simulink model "Base"  (R2023b)
settings: Solver=ode3  StartTime=0.0  StopTime=inf  RelTol=1e-3  EnableMultiTasking=on
PreLoadFcn:
  | addpath(genpath('AS5600_Driver'))
  | addpath(genpath('Servo_Driver'))
  | addpath(genpath('Wattmeter_INA219_Driver'))
libraries: arduinolib x6, arduinosensorlib x2
settings Model: FPTRunName=Active  SimulationMode=external  ExtModeTrigDuration=2  Creator=Rafael  LastModifiedBy=Rafael
settings SolverCC: AlgebraicLoopSolver=TrustRegion  AutoInsertRateTranBlk=on
settings DataIOCC: LimitDataPoints=on  SaveFormat=Array
settings OptimizationCC: ReuseModelBlockBuffer=off  ExpressionDepthLimit=2147483647  LifeSpan=Inf  MaxStackSize=64
settings DebuggingCC: UnderspecifiedInitializationDetection=Classic  MergeDetectMultiDrivingBlocksExec=none  FcnCallInpInsideContextMsg=warning  UnconnectedInputMsg=warning  UnconnectedOutputMsg=warning  UnconnectedLineMsg=warning  AllowSymbolicDim=off  StateNameClashWarn=warning  SFUnexpectedBacktrackingDiag=warning  SFNoUnconditionalDefaultTransitionDiag=warning  SFExecutionAtInitializationDiag=none  ArithmeticOperatorsInVariantConditions=warning
settings HardwareCC: ProdBitPerPointer=32  ProdBitPerSizeT=32  ProdBitPerPtrDiffT=32  ProdLargestAtomicInteger=Long  ProdLargestAtomicFloat=Double  ProdWordSize=32  ProdHWDeviceType=ARM Compatible->ARM Cortex
settings ModelReferenceCC: EnableRefExpFcnMdlSchedulingChecks=on  PropagateSignalLabelsOutOfModel=off
settings SFSimCC: SimUseLocalCustomCode=off  CustomCodeUndefinedFunction=UseInterfaceOnly
settings RTWCC: Description=Embedded Coder  SystemTargetFile=ert.tlc  HardwareBoard=Arduino Due  TemplateMakefile=ert_default_tmf  GenerateReport=on  RTWVerbose=off  RTWUseLocalCustomCode=off  Toolchain=Arduino ARM  BuildConfiguration=Faster Runs  LaunchReport=on
settings CodeAppCC: ForceParamTrailComments=on  OperatorAnnotations=on  StateflowObjectComments=on  MATLABSourceComments=on
settings ERTTargetCC: MultiwordLength=2048  ERTCustomFileBanners=off  SupportContinuousTime=on  SupportNonInlinedSFcns=on  RemoveResetFunc=off  SupportVariableSizeSignals=on  ModelStepFunctionPrototypeControlCompliant=off  ExtMode=on  ExtModeTransport=3  ExtModeStaticAlloc=on  ExtModeAutomaticAllocSize=off  ExtModeStaticAllocSize=24576  ExtModeMexFile=ext_xcp  ExtModeMexArgs=0 4 115200  ExtModeIntrfLevel=Level2 - Open
settings ConfigComp: CovMetricSettings=dw  CovSaveCumulativeToWorkspaceVar=on  CovSaveSingleToWorkspaceVar=on  CovExternalEMLEnable=off  CovSFcnEnable=off

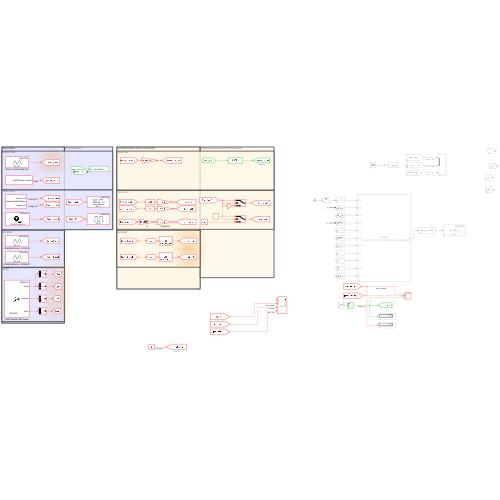
[thumbnail: Simulink's stored preview of the top-level diagram]
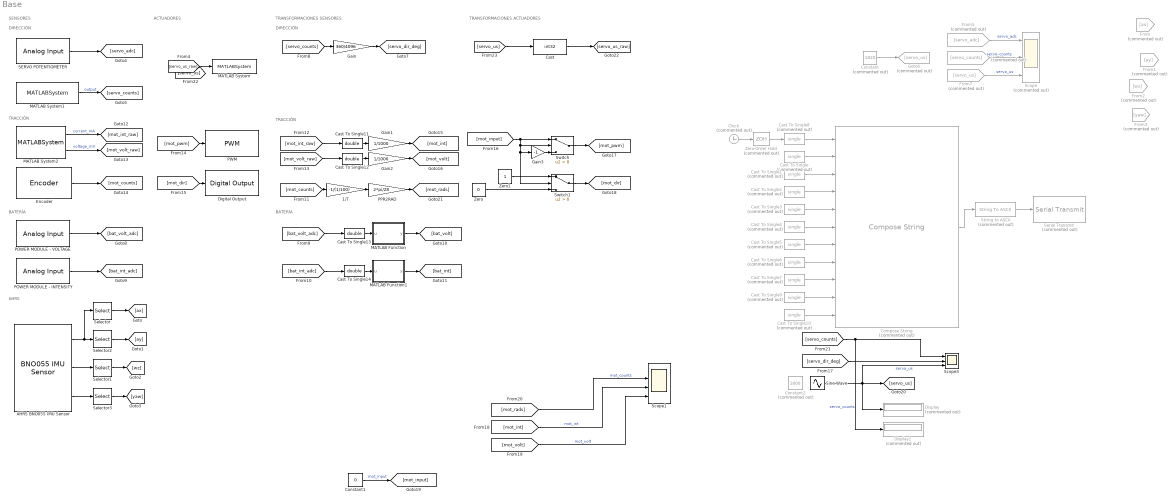
== system Base ==
  note: AHRS
  note: TRACCIÓN
  note: BATERÍA
  note: DIRECCIÓN
  note: ACTUADORES
  note: SENSORES
  note: TRANSFORMACIONES ACTUADORES
  note: TRANSFORMACIONES SENSORES
  note: DIRECCIÓN
  note: BATERÍA
  note: TRACCIÓN
  1/T : Gain  Gain=-1/(1/100)
  AHRS BNO055 IMU Sensor : arduinosensorlib/BNO055 IMU Sensor  SlaveAddress=0x28  OperationMode=Fusion  Accel=on  AngularRate=on  MagField=off  EulerAngles=on  Quat=off  LinearAccel=off  GravityVector=off  Status=off  Timestamp=off  AccelRange=4G  AccelBW=62.5 Hz  GyroRange=2000 dps  GyroBW=32 Hz  MagODR=10 Hz  spf=1  SampleTime=1/100  blockPlatform=ARDUINO  QueueSizeFactor=1
  Cast : DataTypeConversion  OutDataTypeStr=int32  SaturateOnIntegerOverflow=off  RndMeth=Floor
  Cast To Single{,1..10} (11 alike) : DataTypeConversion  Commented=on  OutDataTypeStr=single  SaturateOnIntegerOverflow=off  RndMeth=Floor
  Cast To Single{11..14} (4 alike) : DataTypeConversion  OutDataTypeStr=double  SaturateOnIntegerOverflow=off  RndMeth=Floor
  Clock : Clock  Commented=on
      settings: Decimation=3
  Compose String : ComposeString  Commented=on  Format="\"A,%.3f,%.2f,%.2f,%.2f,%.2f,%.2f,%.2f,%.2f,%.2f,%.2f,%.2f,Z\\n\""
  Constant : Constant  Commented=on  Value=1820  OutDataTypeStr=int32  SampleTime=1/50
  Constant1 : Constant  Value=0  SampleTime=1/100
  Constant2 : Constant  Commented=on  Value=1800  OutDataTypeStr=int32  SampleTime=1/100
  Digital Output : arduinolib/Digital Output  pinNumber=6  Direction=output  blockPlatform=arduino
  Display : Display  Commented=on
  Display1 : Display  Commented=on
  Encoder : arduinosensorlib/Encoder  InputA=2  InputB=3  Mode=Reset at each Sample time  SampleTime=1/100
  From : From  Commented=on  GotoTag=ax
  From1 : From  Commented=on  GotoTag=ay
  From2 : From  Commented=on  GotoTag=wz
  From3 : From  Commented=on  GotoTag=yaw
  From5 : From  Commented=on  GotoTag=servo_adc
  From6 : From  Commented=on  GotoTag=servo_counts
  From7 : From  Commented=on  GotoTag=servo_us
  Gain : Gain  Gain=360/4096
  Gain1 : Gain  Gain=1/1000
  Gain2 : Gain  Gain=1/1000
  Gain3 : Gain  Gain=-1
  Goto6 : Goto  Commented=on  GotoTag=servo_us
  MATLAB Function : MATLAB Function  TreatAsAtomicUnit=on
  MATLAB Function1 : MATLAB Function  TreatAsAtomicUnit=on
  MATLAB System : MATLABSystem  System=ServoDriver  pin=5  min_us=1000  max_us=2500  SampleTime=1/50
      mask Type: ServoDriver
      mask Display:
      | disp('ServoDriver');
      | port_label('input',1,'us');
  MATLAB System1 : MATLABSystem  System=AS5600Driver  SampleTime=0.01
      mask Type: AS5600Driver
      mask Display:
      | disp('AS5600Driver');
      | port_label('output',1,'counts');
  MATLAB System2 : MATLABSystem  System=WattmeterINA219Driver  id=0  wire_number=1  address=45  SampleTime=1/100
      mask Type: WattmeterINA219Driver
      mask Display:
      | disp('WattmeterINA219Driver');
      | port_label('output',1,'current_mA');
      | port_label('output',2,'voltage_mV');
  POWER MODULE - INTENSITY : arduinolib/Analog Input  pinNumber=2  ReadResultsOnly=off  ConversionTriggerSource=Software  ExternalTriggerType=uint32( 0 )  OutputDataType=uint16  EnableConversionCompleteNotify=off  EnableOuputStatus=off  SampleTime=1/100  blockPlatform=arduino
  POWER MODULE - VOLTAGE : arduinolib/Analog Input  pinNumber=1  ReadResultsOnly=off  ConversionTriggerSource=Software  ExternalTriggerType=uint32( 0 )  OutputDataType=uint16  EnableConversionCompleteNotify=off  EnableOuputStatus=off  SampleTime=1/100  blockPlatform=arduino
  PPR2RAD : Gain  Gain=2*pi/28
  PWM : arduinolib/PWM  pinNumber=7  frequencyType=Default  desiredFrequency=490.2  achievableFrequency=490.2
  SERVO POTENTIOMETER : arduinolib/Analog Input  pinNumber=0  ReadResultsOnly=off  ConversionTriggerSource=Software  ExternalTriggerType=uint32( 0 )  OutputDataType=uint16  EnableConversionCompleteNotify=off  EnableOuputStatus=off  SampleTime=1/100  blockPlatform=arduino
  Scope : Scope  Commented=on  NumInputPorts=3
  Scope1 : Scope  NumInputPorts=4
  Scope3 : Scope  NumInputPorts=3
  Selector : Selector  InputPortWidth=3  IndexOptions=Index vector (dialog)  Indices=[1]  OutputSizes=1
  Selector1 : Selector  InputPortWidth=3  IndexOptions=Index vector (dialog)  Indices=[3]  OutputSizes=1
  Selector2 : Selector  InputPortWidth=3  IndexOptions=Index vector (dialog)  Indices=[2]  OutputSizes=1
  Selector3 : Selector  InputPortWidth=3  IndexOptions=Index vector (dialog)  Indices=[3]  OutputSizes=1
  Serial Transmit : arduinolib/Serial Transmit  Commented=on  portNumber=1  sendmode=write  sendformat=Decimal  floatprecision=2  blockPlatform=arduino
  Sine Wave : Sin  Amplitude=400  Bias=1800  Frequency=0.1  SampleTime=1/50
  String to ASCII : StringToASCII  Commented=on  OutputVectorSize=64
  Switch : Switch  Criteria=u2 > Threshold  SaturateOnIntegerOverflow=off  InputSameDT=off
  Switch1 : Switch  Criteria=u2 > Threshold  SaturateOnIntegerOverflow=off  InputSameDT=off
  Zero : Constant  Value=0  OutDataTypeStr=Inherit: Inherit via back propagation  SampleTime=1/100
  Zero-Order Hold : ZeroOrderHold  Commented=on  SampleTime=1/100
  Zero1 : Constant  OutDataTypeStr=Inherit: Inherit via back propagation  SampleTime=1/100
  wires:
  ? -> Cast To Single/1
  Cast To Single6/1 -> Compose String/8
  Cast To Single2/1 -> Compose String/4
  Zero-Order Hold/1 -> Cast To Single8/1
  Cast To Single5/1 -> Compose String/7
  Clock/1 -> Zero-Order Hold/1
  Cast To Single1/1 -> Compose String/3
  ? -> Cast To Single2/1
  String to ASCII/1 -> Serial Transmit/1
  Cast To Single4/1 -> Compose String/6
  Compose String/1 -> String to ASCII/1
  Cast To Single3/1 -> Compose String/5
  Cast To Single/1 -> Compose String/2
  Cast To Single7/1 -> Compose String/9
  Cast To Single8/1 -> Compose String/1
  Selector3/1 -> [yaw]
  AHRS BNO055 IMU Sensor/3 -> Selector3/1
  AHRS BNO055 IMU Sensor/2 -> Selector1/1
  AHRS BNO055 IMU Sensor/1 -> Selector2/1, Selector/1
  Selector2/1 -> [ay]
  Cast To Single9/1 -> Compose String/10
  Cast To Single10/1 -> Compose String/11
  Selector/1 -> [ax]
  Selector1/1 -> [wz]
  SERVO POTENTIOMETER/1 -> [servo_adc]
  MATLAB System1/1 -> [servo_counts]  "output"
  [servo_us_raw] -> MATLAB System/1
  From5/1 -> Scope/1  "servo_adc"
  From6/1 -> Scope/2  "servo_counts"
  From7/1 -> Scope/3  "servo_us"
  Constant/1 -> Goto6/1
  [servo_counts] -> Gain/1
  Gain/1 -> [servo_dir_deg]
  Encoder/1 -> [mot_counts]
  POWER MODULE - VOLTAGE/1 -> [bat_volt_adc]
  POWER MODULE - INTENSITY/1 -> [bat_int_adc]
  [bat_volt_adc] -> Cast To Single13/1
  MATLAB Function/1(y) -> [bat_volt]
  MATLAB System2/1 -> [mot_int_raw]  "current_mA"
  MATLAB System2/2 -> [mot_volt_raw]  "voltage_mV"
  [mot_pwm] -> PWM/1
  [mot_dir] -> Digital Output/1
  Cast To Single13/1 -> MATLAB Function/1(u)
  [mot_rads] -> Scope1/2  "mot_counts"
  [mot_int] -> Scope1/3  "mot_int"
  [mot_volt] -> Scope1/4  "mot_volt"
  Sine Wave/1 -> Display/1, Scope3/3, [servo_us]  "servo_us"
  [servo_dir_deg] -> Scope3/2
  [servo_counts] -> Display1/1, Scope3/1  "servo_counts"
  [servo_us] -> Cast/1
  Cast/1 -> [servo_us_raw]
  Gain2/1 -> [mot_volt]
  [mot_input] -> Switch/1, Switch/2, Switch1/2, Gain3/1
  Cast To Single12/1 -> Gain2/1
  MATLAB Function1/1(y) -> [bat_int]
  [mot_volt_raw] -> Cast To Single12/1
  [mot_int_raw] -> Cast To Single11/1
  [bat_int_adc] -> Cast To Single14/1
  PPR2RAD/1 -> [mot_rads]
  Gain1/1 -> [mot_int]
  Switch/1 -> [mot_pwm]
  Cast To Single14/1 -> MATLAB Function1/1(u)
  Gain3/1 -> Switch/3
  Zero1/1 -> Switch1/1
  Switch1/1 -> [mot_dir]
  Constant1/1 -> [mot_input]  "mot_input"
  Cast To Single11/1 -> Gain1/1
  1/T/1 -> PPR2RAD/1
  [mot_counts] -> 1/T/1
  Zero/1 -> Switch1/3

== matlab function Base/MATLAB Function ==
  data: u input; y output
function y = calib_bat_volt(u)

y = 121.87 * u + 5.03;

if y < 0
    y = 0;
end

== matlab function Base/MATLAB Function1 ==
  data: u input; y output
function y = calib_bat_int(u)

y = 62.77 * u - 11.89;

if y < 0
    y = 0;
end
